simulink model "misc_blocks_Voltage_sag"  (R2025a)
settings: Solver=VariableStepAuto  StartTime=0.0  StopTime=10.0  RelTol=1e-3
undefined symbols (not defined in the file): Nbuses
settings Model: Creator=atomas  LastModifiedBy=atomas

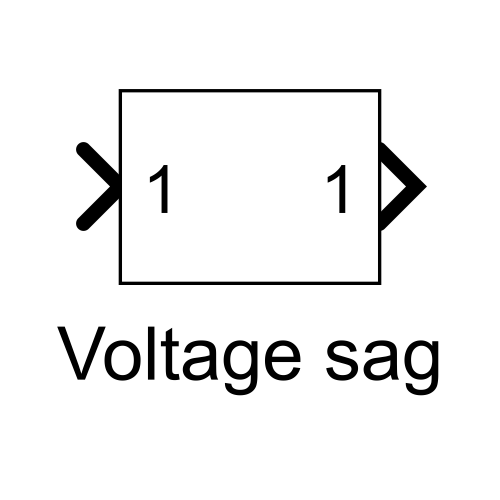
[thumbnail: Simulink's stored preview of the top-level diagram]
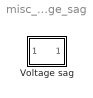
== system misc_blocks_Voltage_sag ==
  Voltage sag : Subsystem

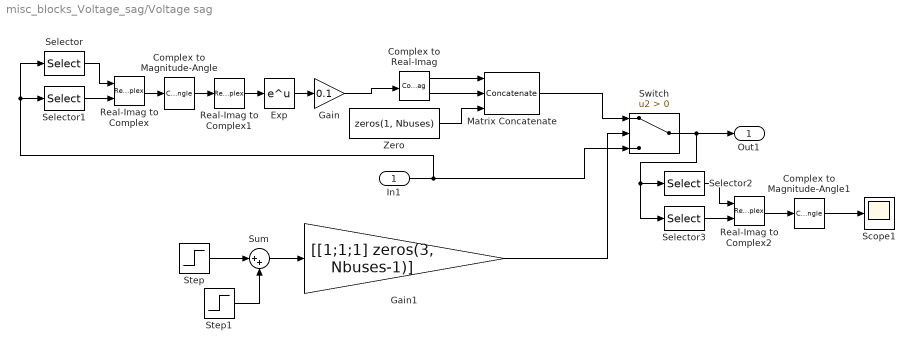
== system misc_blocks_Voltage_sag/Voltage sag ==
  In1 : Inport
  Complex to Magnitude-Angle : ComplexToMagnitudeAngle  Output=Angle
  Complex to Magnitude-Angle1 : ComplexToMagnitudeAngle  Output=Magnitude
  Complex to Real-Imag : ComplexToRealImag
  Exp : Math
  Gain : Gain  Gain=0.1
  Gain1 : Gain  Gain=[[1;1;1] zeros(3, Nbuses-1)]
  Matrix Concatenate : Concatenate  NumInputs=3  Mode=Multidimensional array
  Real-Imag to Complex : RealImagToComplex
  Real-Imag to Complex1 : RealImagToComplex  Input=Imag
  Real-Imag to Complex2 : RealImagToComplex
  Scope1 : Scope
      settings: ActiveDisplayYMinimum=-1  ActiveDisplayYMaximum=1  DataLoggingVariableName=ScopeData2
  Selector : Selector  NumberOfDimensions=2  InputPortWidth=3  IndexOptions=Index vector (dialog),Select all  Indices=1,1  OutputSizes=1,1
  Selector1 : Selector  NumberOfDimensions=2  InputPortWidth=3  IndexOptions=Index vector (dialog),Select all  Indices=2,1  OutputSizes=1,1
  Selector2 : Selector  NumberOfDimensions=2  InputPortWidth=3  IndexOptions=Index vector (dialog),Select all  Indices=1,1  OutputSizes=1,1
  Selector3 : Selector  NumberOfDimensions=2  InputPortWidth=3  IndexOptions=Index vector (dialog),Select all  Indices=2,1  OutputSizes=1,1
  Step : Step  SampleTime=0  VectorParams1D=off
  Step1 : Step  Time=1.05  After=-1  SampleTime=0  VectorParams1D=off
  Sum : Sum  Inputs=|++
  Switch : Switch  Criteria=u2 > Threshold  SaturateOnIntegerOverflow=off  InputSameDT=off
  Zero : Constant  Value=zeros(1, Nbuses)  VectorParams1D=off  OutDataTypeStr=Inherit: Inherit via back propagation
  Out1 : Outport
  wires:
  Step1/1 -> Sum/2
  Sum/1 -> Gain1/1
  Step/1 -> Sum/1
  Complex to Magnitude-Angle1/1 -> Scope1/1
  Real-Imag to Complex2/1 -> Complex to Magnitude-Angle1/1
  Selector2/1 -> Real-Imag to Complex2/1
  Selector3/1 -> Real-Imag to Complex2/2
  Switch/1 -> Out1/1, Selector2/1, Selector3/1
  Gain/1 -> Complex to Real-Imag/1
  Complex to Real-Imag/2 -> Matrix Concatenate/2
  Complex to Real-Imag/1 -> Matrix Concatenate/1
  Zero/1 -> Matrix Concatenate/3
  Matrix Concatenate/1 -> Switch/1
  Real-Imag to Complex1/1 -> Exp/1
  Complex to Magnitude-Angle/1 -> Real-Imag to Complex1/1
  In1/1 -> Selector1/1, Selector/1, Switch/3
  Selector1/1 -> Real-Imag to Complex/2
  Selector/1 -> Real-Imag to Complex/1
  Real-Imag to Complex/1 -> Complex to Magnitude-Angle/1
  Exp/1 -> Gain/1
  Gain1/1 -> Switch/2
